simulink model "example"  (R2012b)
settings: Solver=FixedStepDiscrete  StartTime=0.0  StopTime=inf  RelTol=1e-3
libraries: MAVLink_Block x1
settings Model: Creator=fede  LastModifiedBy=fede

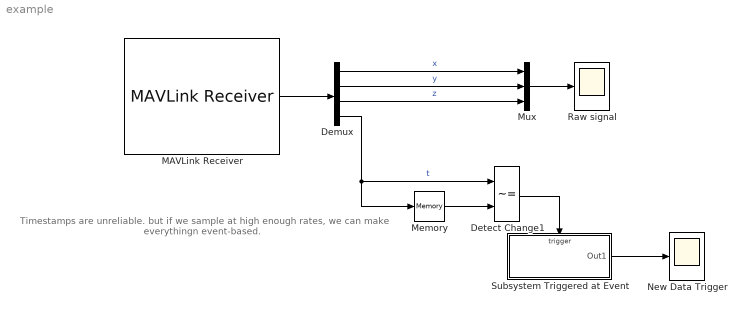
== system example ==
  note: Timestamps are unreliable. but if we
      | sample at high enough rates, we
      | can make everythingn event-based.
  Demux : Demux
  Detect Change1 : RelationalOperator  Operator=~=  OutDataTypeStr=boolean
  MAVLink Receiver : MAVLink_Block/MAVLink Receiver  Port=14550  FS=0.01  accel=off  gyro=on  magn=off  vispos=off  visatt=off  msg_vector=0
  Memory : Memory
  Mux : Mux  Inputs=3
  New Data Trigger : Scope
      settings: ShowLegends=on  TimeRange=5000  YMin=-0.25  YMax=1.25  MaxDataPoints=25000
  Raw signal : Scope
      settings: ShowLegends=on  TimeRange=5000  YMin=-2.5  YMax=1.75  MaxDataPoints=25000
  Subsystem Triggered at Event : Subsystem  TreatAsAtomicUnit=on
  wires:
  MAVLink Receiver/1 -> Demux/1
  Mux/1 -> Raw signal/1
  Demux/1 -> Mux/1  "x"
  Demux/2 -> Mux/2  "y"
  Demux/3 -> Mux/3  "z"
  Demux/4 -> Memory/1, Detect Change1/1  "t"
  Memory/1 -> Detect Change1/2
  Detect Change1/1 -> Subsystem Triggered at Event/Trigger
  Subsystem Triggered at Event/1(Out1) -> New Data Trigger/1

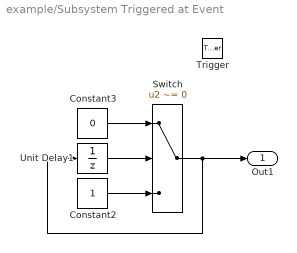
== system example/Subsystem Triggered at Event ==
  Trigger : TriggerPort
  Constant2 : Constant
  Constant3 : Constant  Value=0
  Switch : Switch  Criteria=u2 ~= 0
  Unit Delay1 : UnitDelay  SampleTime=-1
  Out1 : Outport  InitialOutput=0
  wires:
  Constant3/1 -> Switch/1
  Constant2/1 -> Switch/3
  Unit Delay1/1 -> Switch/2
  Switch/1 -> Out1/1, Unit Delay1/1
